simulink model "test09"  (R2021a)
settings: Solver=VariableStepAuto  StartTime=0.0  StopTime=8  RelTol=1e-3
libraries: HORTISIM x3
settings Model: Creator=djoroya  LastModifiedBy=djoroya
settings DebuggingCC: UnconnectedInputMsg=none  UnconnectedOutputMsg=none  UnconnectedLineMsg=none

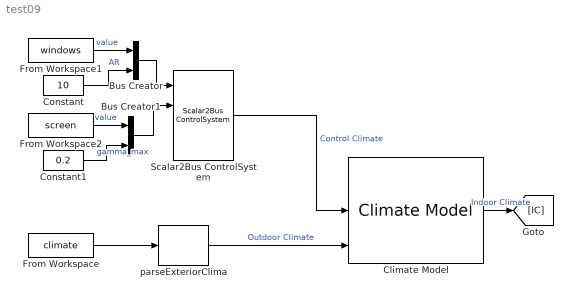
== system test09 ==
  Bus Creator : BusCreator  Inputs=2
  Bus Creator1 : BusCreator  Inputs=2
  Climate Model : HORTISIM/Climate/Models/Climate Model  params=params  x0=cic
      settings: SourceProductName=Horti Simulator
  Constant : Constant  Value=10
  Constant1 : Constant  Value=0.2
  From Workspace : FromWorkspace  VariableName=climate
  From Workspace1 : FromWorkspace  VariableName=windows
  From Workspace2 : FromWorkspace  VariableName=screen
  Scalar2Bus ControlSystem : HORTISIM/Other  Functions/Scalar2Bus  ControlSystem  SystemSampleTime=-1  VariantActivationTime=update diagram  Latency=0  AutoFrameSizeCalculation=off
      settings: SourceProductName=Horti Simulator
  parseExteriorClima : HORTISIM/Other  Functions/parseExteriorClima  SystemSampleTime=-1  VariantActivationTime=update diagram  Latency=0  AutoFrameSizeCalculation=off
      settings: SourceProductName=Horti Simulator
  wires:
  From Workspace/1 -> parseExteriorClima/1
  parseExteriorClima/1 -> Climate Model/3  "Outdoor Climate"
  Climate Model/1 -> [IC]  "Indoor Climate"
  Scalar2Bus ControlSystem/1 -> Climate Model/2  "Control Climate"
  From Workspace1/1 -> Bus Creator/1  "value"
  Constant/1 -> Bus Creator/2  "AR"
  Bus Creator/1 -> Scalar2Bus ControlSystem/1
  From Workspace2/1 -> Bus Creator1/1  "value"
  Constant1/1 -> Bus Creator1/2  "gamma_max"
  Bus Creator1/1 -> Scalar2Bus ControlSystem/2
